simulink model "sat_dyn_simscape"  (R2021b)
settings: Solver=VariableStepAuto  StartTime=0.0  StopTime=10.0  RelTol=1e-3  AbsTol=1e-3  EnableMultiTasking=on
libraries: sharedtransform x2, dynamics_lib x2
settings Model: Creator=DanKvist  LastModifiedBy=DanKvist
settings SolverCC: AutoScaleAbsTol=off  AlgebraicLoopSolver=TrustRegion
settings DataIOCC: LimitDataPoints=on  MaxDataPoints=10000
settings OptimizationCC: LifeSpan=inf
settings DebuggingCC: AllowSymbolicDim=off  SFUnexpectedBacktrackingDiag=warning  SFNoUnconditionalDefaultTransitionDiag=warning  SFExecutionAtInitializationDiag=none  SFMachineParentedDataDiag=warning  ArithmeticOperatorsInVariantConditions=warning
settings SFSimCC: SimUseLocalCustomCode=off  CustomCodeUndefinedFunction=UseInterfaceOnly
settings RTWCC: RTWUseLocalCustomCode=off
settings CodeAppCC: StateflowObjectComments=on
settings GRTTargetCC: TargetLangStandard=C89/C90 (ANSI)
settings ConfigComp: CovMetricSettings=dw  CovSaveCumulativeToWorkspaceVar=on  CovSaveSingleToWorkspaceVar=on  CovExternalEMLEnable=off  CovSFcnEnable=off
settings SimscapeCC: SimscapeLogType=all  SimscapeLogSimulationStatistics=on  SimscapeLogDataHistory=10000

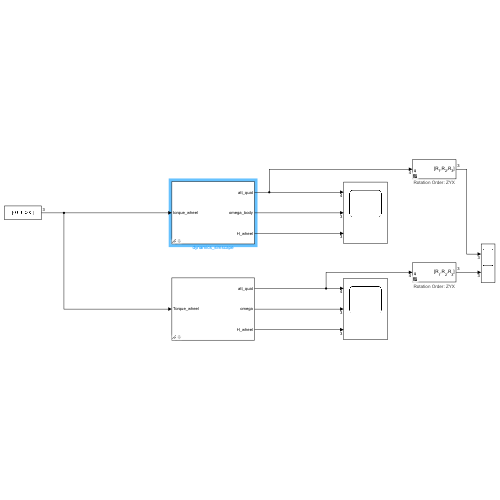
[thumbnail: Simulink's stored preview of the top-level diagram]
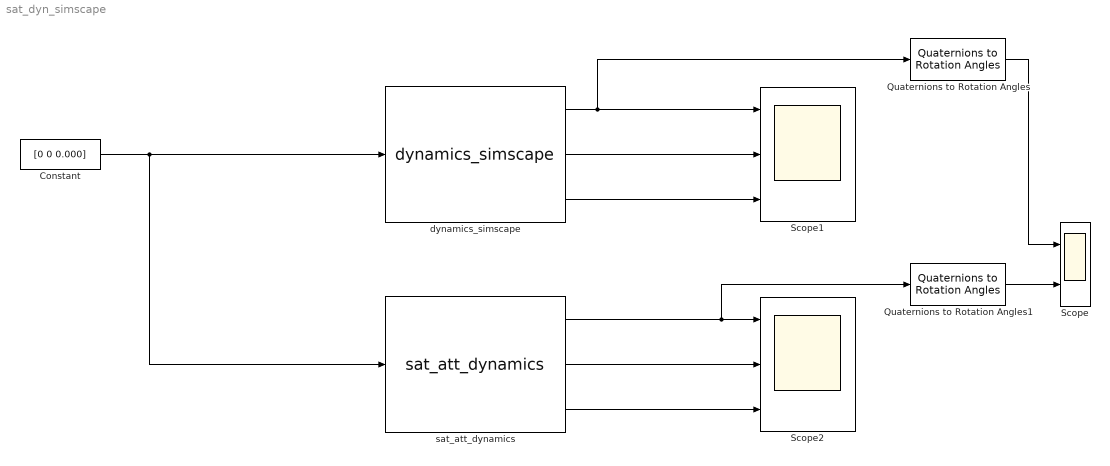
== system sat_dyn_simscape ==
  Constant : Constant  Value=[0 0 0.000]
  Quaternions to Rotation Angles : sharedtransform/Quaternions to Rotation Angles  rotationOrder=ZYX  aMode=aMode
      settings: SourceProductBaseCode=AE,PW,DR,MT,UV,VE
  Quaternions to Rotation Angles1 : sharedtransform/Quaternions to Rotation Angles  rotationOrder=ZYX  aMode=aMode
      settings: SourceProductBaseCode=AE,PW,DR,MT,UV,VE
  Scope : Scope  NumInputPorts=2
  Scope1 : Scope  NumInputPorts=3
  Scope2 : Scope  NumInputPorts=3
  dynamics_simscape : dynamics_lib/dynamics_simscape  I=[1 0 0;0 1 0;0 0 1]  omega_0=[0 0 1]  q_0=[1 0 0 0]  I_w=1.81e-5 * [1 1 1]  torque_wheel_max=0.004 * [1 1 1]  omega_wheel_0=[200 0 0]
  sat_att_dynamics : dynamics_lib/sat_att_dynamics  I=[1 0 0;0 1 0;0 0 1]  omega_0=[0 0 1]  q_0=[1 0 0 0]  I_w=1.81e-5 * [1 1 1]  torque_wheel_max=0.004  momentum_wheel_max=0.015  omega_wheel_0=[200 0 0]
  wires:
  Constant/1 -> sat_att_dynamics/1, dynamics_simscape/1
  dynamics_simscape/3 -> Scope1/3
  dynamics_simscape/1 -> Quaternions to Rotation Angles/1, Scope1/1
  dynamics_simscape/2 -> Scope1/2
  sat_att_dynamics/1 -> Quaternions to Rotation Angles1/1, Scope2/1
  sat_att_dynamics/2 -> Scope2/2
  sat_att_dynamics/3 -> Scope2/3
  Quaternions to Rotation Angles/1 -> Scope/1
  Quaternions to Rotation Angles1/1 -> Scope/2
